simulink model "SMC"  (R2020a)
settings: Solver=ode14x  StartTime=0.0  StopTime=15  FixedStep=1e-3  RelTol=1e-3
values from neighbouring files (symbols this model uses):
  lamda = 600    [script_smc.m]
  lamdast = 850    [script_smc.m]
settings Model: Creator=Admin  LastModifiedBy=Admin
settings DataIOCC: ReturnWorkspaceOutputsName=SMC_out_with

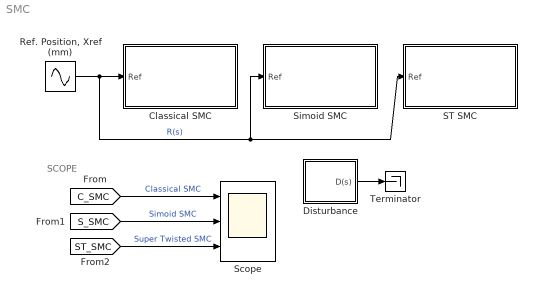
== system SMC ==
  note: SCOPE
  Classical SMC : Subsystem
  Disturbance : Subsystem
  "Ref. Position, Xref (mm)" : Sin  Amplitude=5  Frequency=0.5*(2*pi)  SampleTime=0  Offset=1/2000
  ST SMC : Subsystem
  Scope : Scope  NumInputPorts=3
  Simoid SMC : Subsystem
  Terminator : Terminator
  wires:
  "Ref. Position, Xref (mm)"/1 -> Classical SMC/1(Ref), Simoid SMC/1(Ref), ST SMC/1(Ref)  "R(s)"
  [C_SMC] -> Scope/1  "Classical SMC"
  [S_SMC] -> Scope/2  "Simoid SMC"
  [ST_SMC] -> Scope/3  "Super Twisted SMC"
  Disturbance/1(D(s)) -> Terminator/1

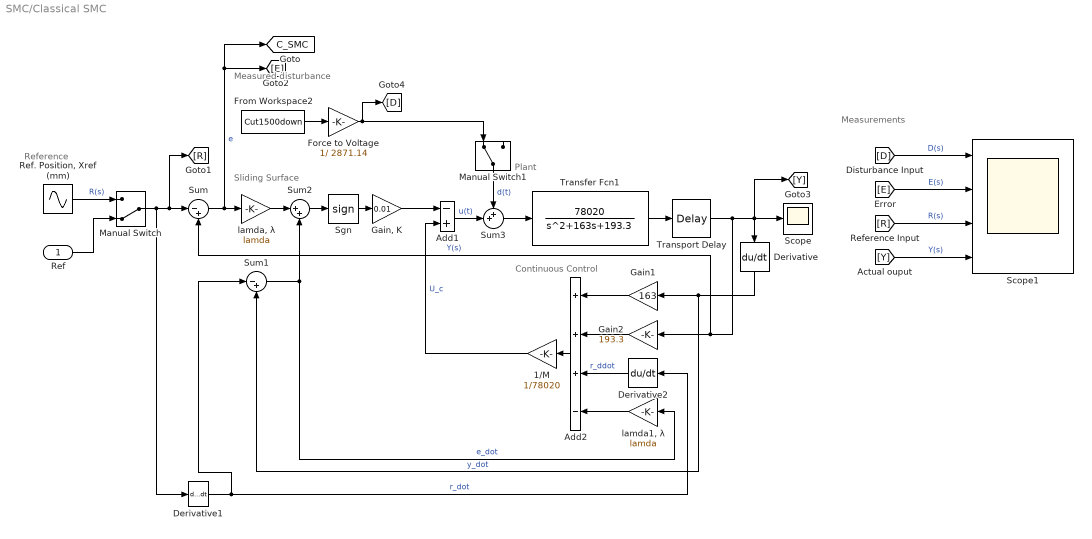
== system SMC/Classical SMC ==
  note: Reference
  note: Sliding Surface
  note: Continuous Control
  note: Measurements
  note: Measured disturbance
  note: Plant
  Ref : Inport
  1/M : Gain  Gain=1/78020
  Add1 : Sum  Inputs=-+
  Add2 : Sum  Inputs=+++-
  Derivative : Derivative
  Derivative1 : Derivative
  Derivative2 : Derivative
  Force to Voltage : Gain  Gain=1/ 2871.14
  From Workspace2 : FromWorkspace  VariableName=Cut1500down  OutDataTypeStr=double  OutputAfterFinalValue=Setting to zero
  "Gain, K" : Gain  Gain=0.01
  Gain1 : Gain  Gain=163
  Gain2 : Gain  Gain=193.3
  Manual Switch : ManualSwitch  CurrentSetting=0
  Manual Switch1 : ManualSwitch
  "Ref. Position, Xref (mm)" : Sin  Amplitude=5  Frequency=0.5*(2*pi)  SampleTime=0  Offset=1/2000
  Scope : Scope
  Scope1 : Scope  NumInputPorts=4
  Sgn : Signum
  Sum : Sum  Inputs=|-+
  Sum1 : Sum  Inputs=|-+
  Sum2 : Sum  Inputs=|++
  Sum3 : Sum  Inputs=++|
  Transfer Fcn1 : TransferFcn  Numerator=[78020]  Denominator=[1 163 193.3]
  Transport Delay : TransportDelay  DelayTime=0.0012
  "lamda, λ" : Gain  Gain=lamda
  "lamda1, λ" : Gain  Gain=lamda
  tag scope: C_SMC=global
  wires:
  Derivative2/1 -> Add2/3  "r_ddot"
  "Gain, K"/1 -> Add1/1
  [E] -> Scope1/2  "E(s)"
  Derivative1/1 -> Derivative2/1, Sum1/1  "r_dot"
  Transport Delay/1 -> [Y], Derivative/1, Scope/1, Gain2/1, Sum/2  "Y(s)"
  [Y] -> Scope1/4  "Y(s)"
  [R] -> Scope1/3  "R(s)"
  [D] -> Scope1/1  "D(s)"
  "Ref. Position, Xref (mm)"/1 -> Manual Switch/1  "R(s)"
  Add1/1 -> Sum3/2  "u(t)"
  1/M/1 -> Add1/2  "U_c"
  Derivative/1 -> Sum1/2, Gain1/1  "y_dot"
  "lamda1, λ"/1 -> Add2/4
  Gain1/1 -> Add2/1
  Sum1/1 -> Sum2/2, "lamda1, λ"/1  "e_dot"
  Sgn/1 -> "Gain, K"/1
  Sum/1 -> [C_SMC], [E], "lamda, λ"/1  "e"
  Add2/1 -> 1/M/1
  Gain2/1 -> Add2/2
  "lamda, λ"/1 -> Sum2/1
  Sum2/1 -> Sgn/1
  Sum3/1 -> Transfer Fcn1/1
  Transfer Fcn1/1 -> Transport Delay/1
  Ref/1 -> Manual Switch/2
  Manual Switch/1 -> Sum/1, [R], Derivative1/1
  Force to Voltage/1 -> Manual Switch1/1, [D]
  From Workspace2/1 -> Force to Voltage/1
  Manual Switch1/1 -> Sum3/1  "d(t)"

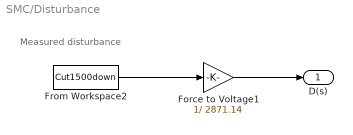
== system SMC/Disturbance ==
  note: Measured disturbance
  Force to Voltage1 : Gain  Gain=1/ 2871.14
  From Workspace2 : FromWorkspace  VariableName=Cut1500down  OutDataTypeStr=double  OutputAfterFinalValue=Setting to zero
  D(s) : Outport
  wires:
  Force to Voltage1/1 -> D(s)/1
  From Workspace2/1 -> Force to Voltage1/1

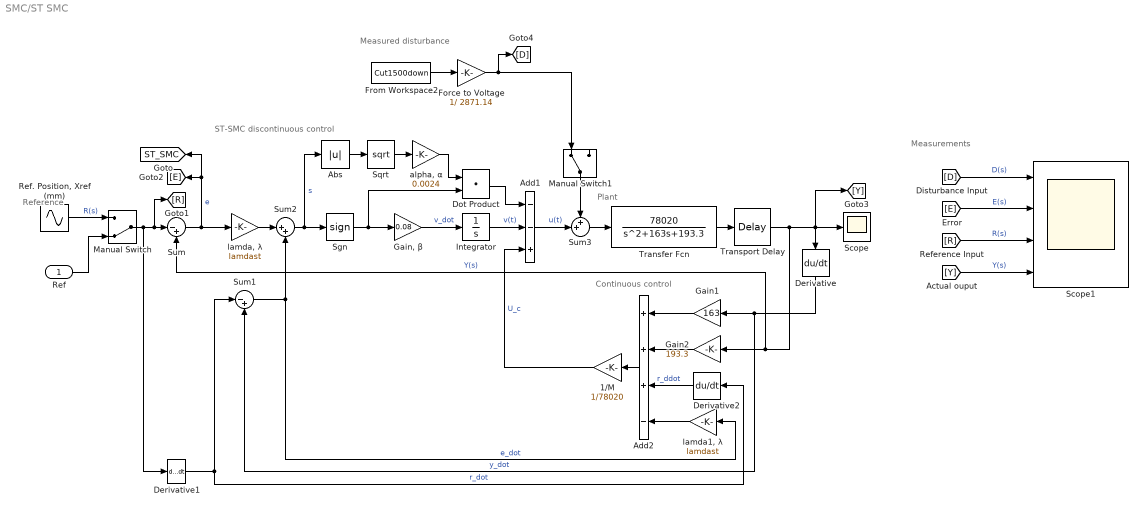
== system SMC/ST SMC ==
  note: Measurements
  note: Measured disturbance
  note: Reference
  note: Plant
  note: ST-SMC discontinuous control
  note: Continuous control
  Ref : Inport
  1/M : Gain  Gain=1/78020
  Abs : Abs
  Add1 : Sum  Inputs=--+
  Add2 : Sum  Inputs=+++-
  Derivative : Derivative
  Derivative1 : Derivative
  Derivative2 : Derivative
  Dot Product : DotProduct  InputSameDT=on  OutDataTypeStr=Inherit: Inherit via internal rule
  Force to Voltage : Gain  Gain=1/ 2871.14
  From Workspace2 : FromWorkspace  VariableName=Cut1500down  OutDataTypeStr=double  OutputAfterFinalValue=Setting to zero
  "Gain, β" : Gain  Gain=0.08
  Gain1 : Gain  Gain=163
  Gain2 : Gain  Gain=193.3
  Integrator : Integrator
  Manual Switch : ManualSwitch  CurrentSetting=0
  Manual Switch1 : ManualSwitch
  "Ref. Position, Xref (mm)" : Sin  Amplitude=5  Frequency=0.5*(2*pi)  SampleTime=0  Offset=1/2000
  Scope : Scope
  Scope1 : Scope  NumInputPorts=4
  Sgn : Signum
  Sqrt : Sqrt  SaturateOnIntegerOverflow=on
  Sum : Sum  Inputs=|-+
  Sum1 : Sum  Inputs=|-+
  Sum2 : Sum  Inputs=|++
  Sum3 : Sum  Inputs=++|
  Transfer Fcn : TransferFcn  Numerator=[78020]  Denominator=[1 163 193.3]
  Transport Delay : TransportDelay  DelayTime=0.0012
  "alpha, α" : Gain  Gain=0.0024
  "lamda, λ" : Gain  Gain=lamdast
  "lamda1, λ" : Gain  Gain=lamdast
  tag scope: ST_SMC=global
  wires:
  Sum3/1 -> Transfer Fcn/1
  Sum2/1 -> Abs/1, Sgn/1  "s"
  "lamda, λ"/1 -> Sum2/1
  Gain2/1 -> Add2/2
  Add2/1 -> 1/M/1
  Sum/1 -> "lamda, λ"/1, [E], [ST_SMC]  "e"
  Sgn/1 -> Dot Product/2, "Gain, β"/1
  Sum1/1 -> Sum2/2, "lamda1, λ"/1  "e_dot"
  Gain1/1 -> Add2/1
  "lamda1, λ"/1 -> Add2/4
  Derivative/1 -> Gain1/1, Sum1/2  "y_dot"
  1/M/1 -> Add1/3  "U_c"
  Add1/1 -> Sum3/2  "u(t)"
  [D] -> Scope1/1  "D(s)"
  [R] -> Scope1/3  "R(s)"
  From Workspace2/1 -> Force to Voltage/1
  [Y] -> Scope1/4  "Y(s)"
  Transfer Fcn/1 -> Transport Delay/1
  Derivative1/1 -> Sum1/1, Derivative2/1  "r_dot"
  [E] -> Scope1/2  "E(s)"
  "Gain, β"/1 -> Integrator/1  "v_dot"
  Force to Voltage/1 -> Manual Switch1/1, [D]
  Derivative2/1 -> Add2/3  "r_ddot"
  Integrator/1 -> Add1/2  "v(t)"
  Abs/1 -> Sqrt/1
  Sqrt/1 -> "alpha, α"/1
  "alpha, α"/1 -> Dot Product/1
  Dot Product/1 -> Add1/1
  Transport Delay/1 -> [Y], Derivative/1, Scope/1, Sum/2, Gain2/1  "Y(s)"
  Manual Switch/1 -> Derivative1/1, Sum/1, [R]
  Ref/1 -> Manual Switch/2
  "Ref. Position, Xref (mm)"/1 -> Manual Switch/1  "R(s)"
  Manual Switch1/1 -> Sum3/1

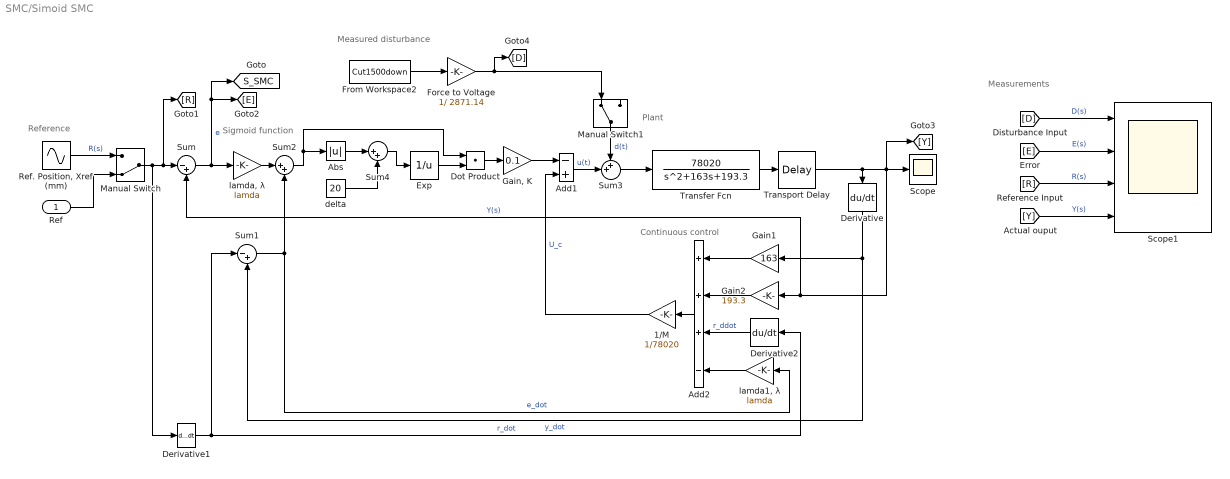
== system SMC/Simoid SMC ==
  note: Sigmoid function
  note: Continuous control
  note: Measurements
  note: Reference
  note: Measured disturbance
  note: Plant
  Ref : Inport
  1/M : Gain  Gain=1/78020
  Abs : Abs
  Add1 : Sum  Inputs=-+
  Add2 : Sum  Inputs=+++-
  Derivative : Derivative
  Derivative1 : Derivative
  Derivative2 : Derivative
  Dot Product : DotProduct  InputSameDT=on  OutDataTypeStr=Inherit: Inherit via internal rule
  Exp : Math  Operator=reciprocal  SaturateOnIntegerOverflow=on
  Force to Voltage : Gain  Gain=1/ 2871.14
  From Workspace2 : FromWorkspace  VariableName=Cut1500down  OutDataTypeStr=double  OutputAfterFinalValue=Setting to zero
  "Gain, K" : Gain  Gain=0.1
  Gain1 : Gain  Gain=163
  Gain2 : Gain  Gain=193.3
  Manual Switch : ManualSwitch  CurrentSetting=0
  Manual Switch1 : ManualSwitch
  "Ref. Position, Xref (mm)" : Sin  Amplitude=5  Frequency=0.5*(2*pi)  SampleTime=0  Offset=1/2000
  Scope : Scope
  Scope1 : Scope  NumInputPorts=4
  Sum : Sum  Inputs=|-+
  Sum1 : Sum  Inputs=|-+
  Sum2 : Sum  Inputs=|++
  Sum3 : Sum  Inputs=++|
  Sum4 : Sum  Inputs=|++
  Transfer Fcn : TransferFcn  Numerator=[78020]  Denominator=[1 163 193.3]
  Transport Delay : TransportDelay  DelayTime=0.0012
  delta : Constant  Value=20
  "lamda, λ" : Gain  Gain=lamda
  "lamda1, λ" : Gain  Gain=lamda
  tag scope: S_SMC=global
  wires:
  Sum3/1 -> Transfer Fcn/1
  "lamda, λ"/1 -> Sum2/1
  Gain2/1 -> Add2/2
  Add2/1 -> 1/M/1
  Sum/1 -> "lamda, λ"/1, [S_SMC], [E]  "e"
  Sum1/1 -> Sum2/2, "lamda1, λ"/1  "e_dot"
  Gain1/1 -> Add2/1
  "lamda1, λ"/1 -> Add2/4
  Derivative/1 -> Gain1/1, Sum1/2  "y_dot"
  1/M/1 -> Add1/2  "U_c"
  Add1/1 -> Sum3/2  "u(t)"
  [D] -> Scope1/1  "D(s)"
  [R] -> Scope1/3  "R(s)"
  From Workspace2/1 -> Force to Voltage/1
  [Y] -> Scope1/4  "Y(s)"
  Transfer Fcn/1 -> Transport Delay/1
  Derivative1/1 -> Sum1/1, Derivative2/1  "r_dot"
  [E] -> Scope1/2  "E(s)"
  Force to Voltage/1 -> Manual Switch1/1, [D]
  Derivative2/1 -> Add2/3  "r_ddot"
  Sum2/1 -> Dot Product/1, Abs/1
  Abs/1 -> Sum4/1
  delta/1 -> Sum4/2
  Sum4/1 -> Exp/1
  Exp/1 -> Dot Product/2
  Dot Product/1 -> "Gain, K"/1
  "Gain, K"/1 -> Add1/1
  Transport Delay/1 -> Scope/1, [Y], Sum/2, Gain2/1, Derivative/1  "Y(s)"
  Manual Switch/1 -> Derivative1/1, Sum/1, [R]
  Ref/1 -> Manual Switch/2
  "Ref. Position, Xref (mm)"/1 -> Manual Switch/1  "R(s)"
  Manual Switch1/1 -> Sum3/1  "d(t)"
